simulink model "Shank_PID_Model"  (R2024b)
settings: Solver=VariableStepAuto  StartTime=0.0  StopTime=80  RelTol=1e-3
values from neighbouring files (symbols this model uses):
  Kd = x(3)    [GA_code.m]    (also in GA_code_Ver2.m; GA_code_Ver3_1_PID.m; Test_GA.m = 28.5419; Test_multi_PID.m = 51.324)
  Ki = x(2)    [GA_code.m]    (also in GA_code_Ver2.m; GA_code_Ver3_1_PID.m; Test_GA.m = 33.8912; Test_multi_PID.m = 199.888)
  Kp = x(1)    [GA_code.m]    (also in GA_code_Ver2.m; GA_code_Ver3_1_PID.m; Test_GA.m = 112.9515; Test_multi_PID.m = 226.746)
  N = x(4)    [GA_code.m]    (also in GA_code_Ver2.m; GA_code_Ver3_1_PID.m; Structures_code_ver1.m = 10000; Test_GA.m = 0)
undefined symbols (not defined in the file or in its folder): DiscIntNeverNeededParam
libraries: slpidlib x1, SignalEditorBlockLib x1, simulink x1
settings Model: Creator=shak2  LastModifiedBy=himma
settings DataIOCC: SaveOutput=off  SignalLogging=off  SaveTime=off

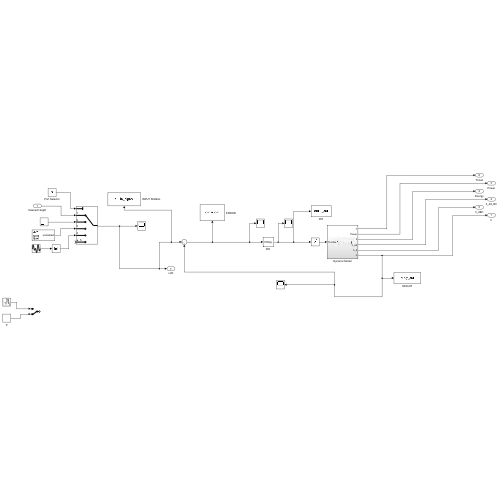
[thumbnail: Simulink's stored preview of the top-level diagram]
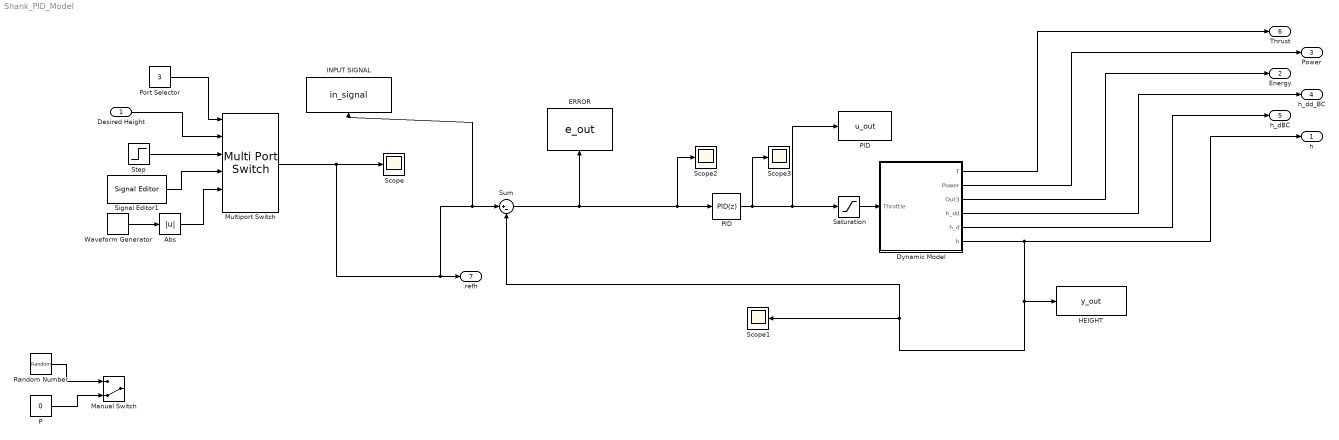
== system Shank_PID_Model ==
  Desired Height : Inport
  Abs : Abs  SaturateOnIntegerOverflow=off
  Dynamic Model : Subsystem
  "ERROR " : ToWorkspace  VariableName=e_out  SaveFormat=Structure With Time  SampleTime=0.05
      settings: Save2DSignal=2-D array (concatenate along first dimension)
  HEIGHT : ToWorkspace  VariableName=y_out  SaveFormat=Structure With Time  SampleTime=0.05
      settings: Save2DSignal=2-D array (concatenate along first dimension)
  INPUT SIGNAL : ToWorkspace  VariableName=in_signal  SaveFormat=Structure With Time  SampleTime=0.05
      settings: Save2DSignal=2-D array (concatenate along first dimension)
  Manual Switch : ManualSwitch  CurrentSetting=0
  Multiport Switch : MultiPortSwitch  Inputs=5  SaturateOnIntegerOverflow=off  InputSameDT=off
  P : Constant  Value=0
  PID : ToWorkspace  VariableName=u_out  SaveFormat=Structure With Time  SampleTime=0.05
      settings: Save2DSignal=2-D array (concatenate along first dimension)
  "PID " : slpidlib/PID Controller  Controller=PID  Form=Parallel  TimeDomain=Discrete-time  UseExternalTs=off  SampleTime=0.05  IntegratorMethod=Forward Euler  FilterMethod=Forward Euler  ControllerParametersSource=internal  P=Kp  I=Ki  UseKiTs=off  D=Kd  UseExternalDerivativeSource=off  N=N  UseFilter=on  TunerSelectOption=Transfer Function Based (PID Tuner App)  InitialConditionSource=internal  InitialConditionForIntegrator=0  InitialConditionForFilter=0  DifferentiatorICPrevScaledInput=0  ExternalReset=none  TrackingMode=off  Kt=1  LimitOutput=off  SatLimitsSource=internal  UpperSaturationLimit=inf  LowerSaturationLimit=-inf  LinearizeAsGain=off  AntiWindupMode=none  Kb=1  LimitIntegrator=off  UpperIntegratorSaturationLimit=inf  LowerIntegratorSaturationLimit=-inf  POutMin=[]  POutMax=[]  IOutMin=[]  IOutMax=[]  DOutMin=[]  DOutMax=[]  NOutMin=[]  NOutMax=[]  SumOutMin=[]  SumOutMax=[]  SaturationOutMin=[]  SaturationOutMax=[]  PParamMin=[]  PParamMax=[]  IParamMin=[]  IParamMax=[]  DParamMin=[]  DParamMax=[]  NParamMin=[]  NParamMax=[]  KbParamMin=[]  KbParamMax=[]  KtParamMin=[]  KtParamMax=[]  KbOutMin=[]  KbOutMax=[]  KtOutMin=[]  KtOutMax=[]  IntegratorOutMin=[]  IntegratorOutMax=[]  FilterOutMin=[]  FilterOutMax=[]  SumI1OutMin=[]  SumI1OutMax=[]  SumI2OutMin=[]  SumI2OutMax=[]  SumI3OutMin=[]  SumI3OutMax=[]  SumI4OutMin=[]  SumI4OutMax=[]  SumDOutMin=[]  SumDOutMax=[]  DifferentiatorOutMin=[]  DifferentiatorOutMax=[]  FilterDiffOutCoefMin=[]  FilterDiffOutCoefMax=[]  ReciprocalOutMin=[]  ReciprocalOutMax=[]  SumDenOutMin=[]  SumDenOutMax=[]  SumNumOutMin=[]  SumNumOutMax=[]  DivideOutMin=[]  DivideOutMax=[]  UdiffTsProdOutMin=[]  UdiffTsProdOutMax=[]  NTsProdOutMin=[]  NTsProdOutMax=[]  UintegralTsProdOutMin=[]  UintegralTsProdOutMax=[]  UngainTsProdOutMin=[]  UngainTsProdOutMax=[]  ClampingZeroOutDataTypeStr=Inherit: Inherit via back propagation  ClampingZeroOutMin=[]  ClampingZeroOutMax=[]  FilterDenConstantOutDataTypeStr=Inherit: Inherit via back propagation  FilterDenConstantOutMin=[]  FilterDenConstantOutMax=[]  PCopyOutDataTypeStr=Inherit: Inherit via back propagation  PCopyOutMin=[]  PCopyOutMax=[]  NCopyOutDataTypeStr=Inherit: Inherit via back propagation  NCopyOutMin=[]  NCopyOutMax=[]  IntegratorContinuousStateAttributes=''  IntegratorStateMustResolveToSignalObject=off  IntegratorRTWStateStorageClass=Auto  FilterContinuousStateAttributes=''  FilterStateMustResolveToSignalObject=off  FilterRTWStateStorageClass=Auto  ParallelPVariant=InternalParameters  IdealPVariant=Disabled  IVariant=InternalParameters  DVariant=InternalParameters  IntegratorVariant=Discrete  SatVariant=Disabled  AWVariant=Passthrough  PCopyVariant=Disabled  TRVariant=Disabled  FdbkBlocksVariant=Forward  IdealPFdbkVariant=Disabled  SatFdbkVariant=Disabled  DerivativeFilterVariant=ForwardEulerFilter  NVariant=InternalParameters  NCopyVariant=Disabled  FilterICVariant=InternalICsFilter  IntegratorICVariant=InternalICs  ExternalResetVariant=Disabled  TRSumVariant=Passthrough  SumFdbkVariant=Disabled  SumVariant=Sum_PID  TsampFilterVariant=InternalTs  TsampNgainVariant=Passthrough  TsampIntegralVariant=Disabled_SignalSpec  ExternalSaturationOutDataTypeStr=Inherit: Same as second input  DerivativeSourceVariant=ErrorSignal  PreIntVariant=InternalPreInt
      settings: LibrarySourceBlock=simulink/Discrete/Discrete PID Controller
  Port Selector : Constant  Value=3
  Random Number : RandomNumber  Variance=0.001  SampleTime=0.1
  Saturation : Saturate  UpperLimit=90  LowerLimit=0
  Scope{,1..3} (4 alike) : Scope
  Signal Editor1 : SignalEditorBlockLib/Signal Editor  FileName=E:\EP2_Summer\Simulink models\ds2.mat  ActiveScenario=ds2  ActiveSignal=unnamed  IsBus=off  OutputBusObjectStr=Bus: BusObject  SampleTime=0  Interpolate=off  ZeroCross=off  OutputAfterFinalValue=Setting to zero  Unit=inherit  PreserveSignalName=on  ApplySigPropsToAllScenarios=on  ApplySigPropsToAllSignals=off
  Step : Step  Time=10  SampleTime=0.05
  Sum : Sum  Inputs=|+-
  Waveform Generator : simulink/Sources/Waveform Generator  OutMin=[]  OutMax=[]  OutDataTypeStr=double  SelectedSignal=1  BlockNames=MultiportSwitch_e3df3653d217406  SampleTime=0.1
  h : Outport
  Energy : Outport  Port=2
  Power : Outport  Port=3
  h_dd_BC : Outport  Port=4
  h_dBC : Outport  Port=5
  Thrust : Outport  Port=6
  refh : Outport  Port=7
  wires:
  Dynamic Model/1(T) -> Thrust/1
  Dynamic Model/2(Power) -> Power/1
  Dynamic Model/3(Out3) -> Energy/1
  Dynamic Model/4(h_dd) -> h_dd_BC/1
  Dynamic Model/5(h_d) -> h_dBC/1
  Saturation/1 -> Dynamic Model/1(Throttle)
  Dynamic Model/6(h) -> HEIGHT/1, Sum/2, Scope1/1, h/1
  Sum/1 -> Scope2/1, "PID "/1, "ERROR "/1
  "PID "/1 -> PID/1, Saturation/1, Scope3/1
  Waveform Generator/1 -> Abs/1
  Abs/1 -> Multiport Switch/5
  Signal Editor1/1 -> Multiport Switch/4
  Step/1 -> Multiport Switch/3
  Desired Height/1 -> Multiport Switch/2
  Port Selector/1 -> Multiport Switch/1
  Random Number/1 -> Manual Switch/1
  Multiport Switch/1 -> Scope/1, Sum/1, INPUT SIGNAL/1, refh/1
  P/1 -> Manual Switch/2

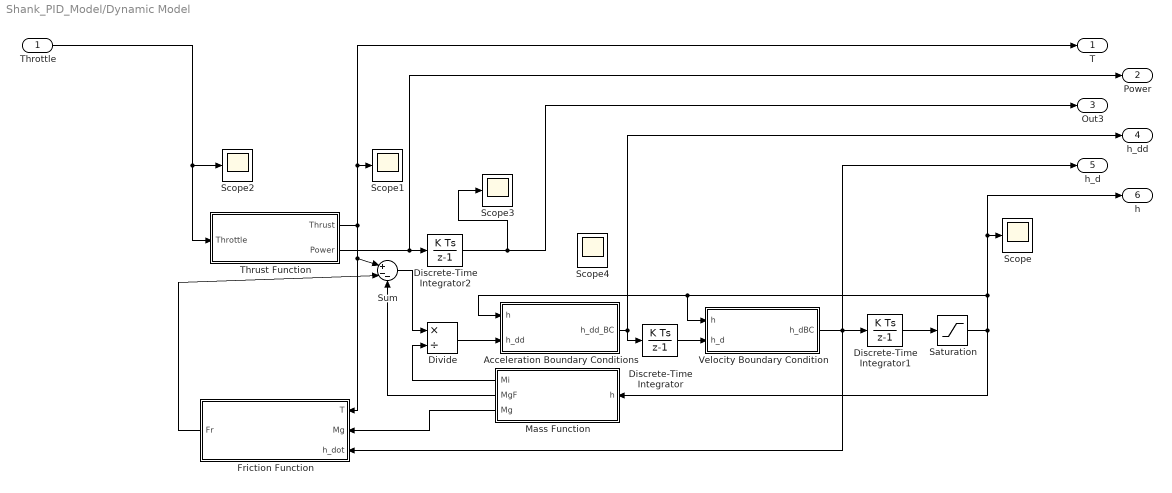
== system Shank_PID_Model/Dynamic Model ==
  Throttle : Inport
  Acceleration Boundary Conditions : MATLAB Function  TreatAsAtomicUnit=on
  Discrete-Time Integrator : DiscreteIntegrator  SampleTime=0.05  ICPrevOutput=DiscIntNeverNeededParam  ICPrevScaledInput=DiscIntNeverNeededParam
  Discrete-Time Integrator1 : DiscreteIntegrator  SampleTime=0.05  ICPrevOutput=DiscIntNeverNeededParam  ICPrevScaledInput=DiscIntNeverNeededParam
  Discrete-Time Integrator2 : DiscreteIntegrator  SampleTime=0.05  ICPrevOutput=DiscIntNeverNeededParam  ICPrevScaledInput=DiscIntNeverNeededParam
  Divide : Product  Inputs=*/
  Friction Function : MATLAB Function  TreatAsAtomicUnit=on
  Mass Function : MATLAB Function  TreatAsAtomicUnit=on
  Saturation : Saturate  UpperLimit=1.44  LowerLimit=0
  Scope{,1..4} (5 alike) : Scope
  Sum : Sum  Inputs=|+--
  Thrust Function : MATLAB Function  TreatAsAtomicUnit=on
  Velocity Boundary Condition : MATLAB Function  TreatAsAtomicUnit=on
  T : Outport
  Power : Outport  Port=2
  Out3 : Outport  Port=3
  h_dd : Outport  Port=4
  h_d : Outport  Port=5
  h : Outport  Port=6
  wires:
  Divide/1 -> Acceleration Boundary Conditions/2(h_dd)
  Velocity Boundary Condition/1(h_dBC) -> h_d/1, Friction Function/3(h_dot), Discrete-Time Integrator1/1
  Saturation/1 -> h/1, Scope/1, Velocity Boundary Condition/1(h), Acceleration Boundary Conditions/1(h), Mass Function/1(h)
  Thrust Function/2(Power) -> Power/1, Discrete-Time Integrator2/1
  Mass Function/1(Mi) -> Divide/2
  Discrete-Time Integrator2/1 -> Scope3/1, Out3/1
  Throttle/1 -> Thrust Function/1(Throttle), Scope2/1
  Thrust Function/1(Thrust) -> T/1, Scope1/1, Friction Function/1(T), Sum/1
  Friction Function/1(Fr) -> Sum/2
  Acceleration Boundary Conditions/1(h_dd_BC) -> h_dd/1, Discrete-Time Integrator/1
  Discrete-Time Integrator/1 -> Velocity Boundary Condition/2(h_d)
  Mass Function/3(Mg) -> Friction Function/2(Mg)
  Mass Function/2(MgF) -> Sum/3
  Discrete-Time Integrator1/1 -> Saturation/1
  Sum/1 -> Divide/1

== matlab function Shank_PID_Model/Dynamic Model/Thrust Function ==
  data: Throttle input; Thrust output; Power output
function [Thrust, Power ]= ThrustFunction(Throttle)

S_t = Throttle/100;

%Throttle to Thrust

% Polyfit 6th Order

a = 0.451880436962741;
b = -1.486027191210204;
c = 1.797219095509746;
d = -0.984318732289241;
e = 0.241341383767270;
f = -0.007579836329288;
g = 0.000042183273304;

Thrust = 2 * (1.0e+03) * (a*S_t^6 + b*S_t^5 + c*S_t^4 + d*S_t^3 + e*S_t^2 + f*S_t + g ); 


% Polyfit 6th Order

a = 1.401054302991919;
b = -4.543527223865324;
c = 5.384918481145972;
d = -2.871958912880594;
e = 0.697342980048495;
f = -0.033090224044331;
g = 0.000320259608978;

Power = 2 * (1.0e+04) * (a*S_t^6 + b*S_t^5 + c*S_t^4 + d*S_t^3 + e*S_t^2 + f*S_t + g );

== matlab function Shank_PID_Model/Dynamic Model/Friction Function ==
  data: T input; Mg input; Fr output; h_dot input
function Fr = FrictionFunction(T, Mg, h_dot)

Cdf = 0.17; %Coefficient of Dynamic Friction

%% geometry *CURRENTLY PLACEHOLDER*
l_t = 0.1; %Thrust Moment Arm
l_cg = 0.05; %CG Moment Arm
l_c = 0.01; %C Moment Arm

if abs(h_dot) == 0
    Fr = 0.26 * 9.81; %static friction
else
    %% THIS IS A PLACEHOLDER
    N = (T * l_t - Mg*9.81*l_cg)/l_c; %Normal reaction force 
    Fr = sign(h_dot)*Cdf*abs(N);
end

== matlab function Shank_PID_Model/Dynamic Model/Acceleration Boundary Conditions ==
  data: h input; h_dd input; h_dd_BC output
function h_dd_BC = Accel_BC(h,h_dd)
% Acceleration must be 0 at the top and bottom
if (h <= 0 && h_dd < 0) || (h >= 1.44 && h_dd > 0)
    h_dd_BC = 0;
else
    h_dd_BC = h_dd;
end

== matlab function Shank_PID_Model/Dynamic Model/Velocity Boundary Condition ==
  data: h input; h_d input; h_dBC output
function h_dBC = Vel_BC(h, h_d)

if (h<=0 && h_d < 0) || (h>=1.44 && h_d > 0)
    h_dBC = 0;
else
    h_dBC = h_d;
end

== matlab function Shank_PID_Model/Dynamic Model/Mass Function ==
  data: Mi output; MgF output; h input; Mg output
function [Mi, MgF, Mg] = MassFunction(h)

%Given Masses in Kg
Mm = 0.328; %Motor Mass
Ma = 0.05; %Arm Mass
Mk = 0.15; %Cart Mass

M_constant = Mm + Mk + Ma;

Mc = 2*(0.095*h + 0.532); %mass of cable is function of height

Mg = M_constant + Mc; %gravitational load
Mi = Mg + 0.8; % gravitational + carriage + counterweight + 8 sliders

MgF = Mg * 9.81;
